simulink model "RLCexample"  (Simulink 7.8)
settings: Solver=ode1  StartTime=0.0  StopTime=10  FixedStep=0.002  RelTol=1e-3
settings Model: Creator=amiria  LastModifiedBy=amiria  ExtModeTrigDuration=5000
settings SolverCC: PositivePriorityOrder=on
settings RTWCC: SystemTargetFile=quarc_win64.tlc  TemplateMakefile=quarc_default_tmf  Description=QUARC Win64 Target  ProcessScript=quarc_win64_make_rtw_hook
settings STFCustomTargetCC: TargetPreCompLibLocation=C:\PROGRA~3\QUARC\lib\2011b\win64\release  SystemTargetFile=quarc_win64.tlc
settings GRTTargetCC: TargetPreCompLibLocation=C:\PROGRA~3\QUARC\lib\2011b\win64\release  ParMdlRefBuildCompliant=off  CompOptLevelCompliant=off  ConcurrentExecutionCompliant=off  MatFileLogging=off  ExtMode=on  ExtModeMexFile=quarc_comm

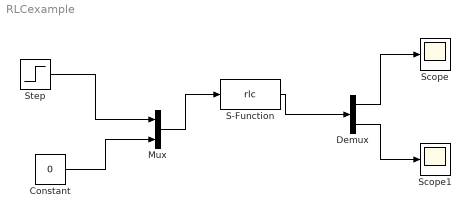
== system RLCexample ==
  Constant : Constant  Value=0
  Demux : Demux  Outputs=2
  Mux : Mux  Inputs=2
  S-Function : S-Function  FunctionName=rlc  EnableBusSupport=off
  Scope : Scope
  Scope1 : Scope
  Step : Step  Time=0  SampleTime=0
  wires:
  S-Function/1 -> Demux/1
  Mux/1 -> S-Function/1
  Demux/1 -> Scope/1
  Demux/2 -> Scope1/1
  Constant/1 -> Mux/2
  Step/1 -> Mux/1
